simulink model "humanFollower2"  (R2018b)
settings: Solver=VariableStepAuto  StartTime=0.0  StopTime=inf  RelTol=1e-3
undefined symbols (not defined in the file or in its folder): Angular, Linear
libraries: robotlib x8
settings Model: Creator=ckreienk  LastModifiedBy=ckreienk

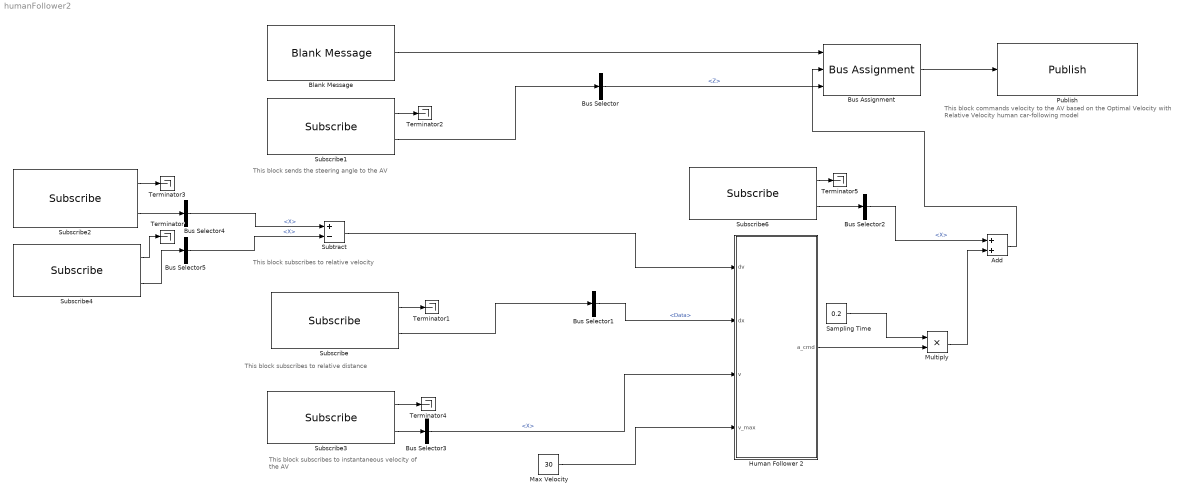
== system humanFollower2 ==
  note: This block sends the steering angle
      | to the AV
  note: This block subscribes to relative velocity
  note: This block subscribes to relative distance
  note: This block subscribes to
      | instantaneous velocity of the AV
  note: This block commands velocity to the AV based
      | on the Optimal Velocity with Relative Velocity
      | human car-following model
  Add : Sum
  Blank Message : robotlib/Blank Message  messageClass=Message  entityType=geometry_msgs/Twist  messageType=geometry_msgs/Twist  SampleTime=inf
      settings: SourceProductBaseCode=RO
  Bus Assignment : BusAssignment  AssignedSignals=Linear.X,Angular.Z
  Bus Selector : BusSelector  OutputSignals=Angular.Z
  Bus Selector1 : BusSelector  OutputSignals=Data
  Bus Selector{2..5} (4 alike) : BusSelector  OutputSignals=Linear.X
  Human Follower 2 : Subsystem
  Max Velocity : Constant  Value=30
  Multiply : Product
  Publish : robotlib/Publish  topicSource=Select from ROS network  topic=/followerVehicle/cmd_vel  messageType=geometry_msgs/Twist  messageQueueLength=1
      settings: SourceProductBaseCode=RO
  Sampling Time : Constant  Value=0.2
  Subscribe : robotlib/Subscribe  topicSource=Select from ROS network  topic=/followerVehicle/distanceEstimatorSteeringBased/dist  messageType=std_msgs/Float64  sampleTime=-1  messageQueueLength=1
      settings: SourceProductBaseCode=RO
  Subscribe1 : robotlib/Subscribe  topicSource=Select from ROS network  topic=/leadVehicle/cmd_vel  messageType=geometry_msgs/Twist  sampleTime=-1  messageQueueLength=1
      settings: SourceProductBaseCode=RO
  Subscribe2 : robotlib/Subscribe  topicSource=Select from ROS network  topic=/leadVehicle/cmd_vel  messageType=geometry_msgs/Twist  sampleTime=-1  messageQueueLength=1
      settings: SourceProductBaseCode=RO
  Subscribe3 : robotlib/Subscribe  topicSource=Select from ROS network  topic=/followerVehicle/cmd_vel  messageType=geometry_msgs/Twist  sampleTime=-1  messageQueueLength=1
      settings: SourceProductBaseCode=RO
  Subscribe4 : robotlib/Subscribe  topicSource=Select from ROS network  topic=/followerVehicle/cmd_vel  messageType=geometry_msgs/Twist  sampleTime=-1  messageQueueLength=1
      settings: SourceProductBaseCode=RO
  Subscribe6 : robotlib/Subscribe  topicSource=Select from ROS network  topic=/followerVehicle/cmd_vel  messageType=geometry_msgs/Twist  sampleTime=-1  messageQueueLength=1
      settings: SourceProductBaseCode=RO
  Subtract : Sum  Inputs=+-
  Terminator{,1..5} (6 alike) : Terminator
  wires:
  Bus Selector2/1 -> Add/1  "<X>"
  Subscribe6/2 -> Bus Selector2/1
  Multiply/1 -> Add/2
  Sampling Time/1 -> Multiply/1
  Human Follower 2/1(a_cmd) -> Multiply/2
  Add/1 -> Bus Assignment/2
  Subscribe6/1 -> Terminator5/1
  Subscribe1/2 -> Bus Selector/1
  Blank Message/1 -> Bus Assignment/1
  Bus Assignment/1 -> Publish/1
  Subscribe/1 -> Terminator1/1
  Subscribe/2 -> Bus Selector1/1
  Subscribe1/1 -> Terminator2/1
  Subscribe2/1 -> Terminator3/1
  Subscribe3/1 -> Terminator4/1
  Subscribe3/2 -> Bus Selector3/1
  Bus Selector1/1 -> Human Follower 2/2(dx)  "<Data>"
  Bus Selector3/1 -> Human Follower 2/3(v)  "<X>"
  Bus Selector/1 -> Bus Assignment/3  "<Z>"
  Subscribe4/1 -> Terminator/1
  Subtract/1 -> Human Follower 2/1(dv)
  Subscribe2/2 -> Bus Selector4/1
  Bus Selector4/1 -> Subtract/1  "<X>"
  Subscribe4/2 -> Bus Selector5/1
  Bus Selector5/1 -> Subtract/2  "<X>"
  Max Velocity/1 -> Human Follower 2/4(v_max)

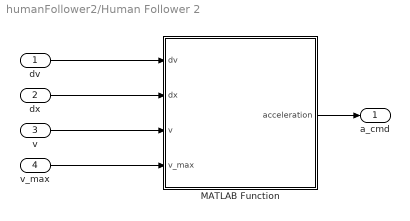
== system humanFollower2/Human Follower 2 ==
  dv : Inport
  dx : Inport  Port=2
  v : Inport  Port=3
  v_max : Inport  Port=4
  MATLAB Function : MATLAB Function  TreatAsAtomicUnit=on
  a_cmd : Outport
  wires:
  dx/1 -> MATLAB Function/2(dx)
  dv/1 -> MATLAB Function/1(dv)
  v/1 -> MATLAB Function/3(v)
  MATLAB Function/1(acceleration) -> a_cmd/1
  v_max/1 -> MATLAB Function/4(v_max)

== matlab function humanFollower2/Human Follower 2/MATLAB Function ==
  data: dv input; dx input; v input; v_max input; acceleration output
function acceleration = fcn(dv, dx, v, v_max)

if dx <= 10
    V = 0;
elseif dx <= 35
    V = dx - 10;
else
    V = 30;
end

if dv + v <= v_max
    w = v + dv;
else
    w = v_max;
end

acceleration = 0.1*(V-v) + 0.5*(w-v);
